simulink model "TSCLAB_Modelv_15_2020a"  (R2020a)
settings: Solver=VariableStepAuto  StartTime=0.0  StopTime=200  RelTol=1e-3
undefined symbols (not defined in the file): LF, serial
libraries: instrumentlib x3
settings Model: Creator=vasanza  LastModifiedBy=victo

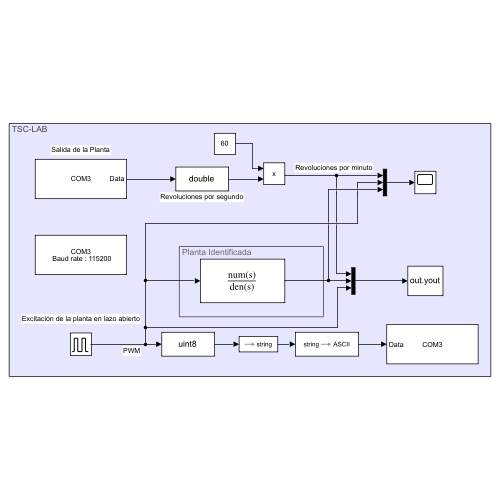
[thumbnail: Simulink's stored preview of the top-level diagram]
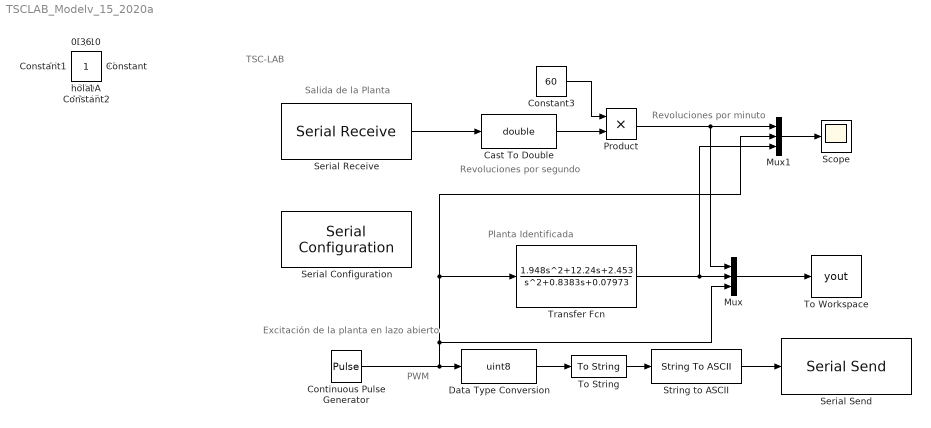
== system TSCLAB_Modelv_15_2020a ==
  note: PWM
  note: Excitación de la planta en lazo abierto
  note: Planta Identificada
  note: Revoluciones por minuto
  note: Revoluciones por segundo
  note: Salida de la Planta
  note: TSC-LAB
  Cast To Double : DataTypeConversion  OutDataTypeStr=double
  Constant3 : Constant  Value=60
  Continuous Pulse Generator : DiscretePulseGenerator  PulseType=Time based  Amplitude=255  Period=24  PulseWidth=50
  Data Type Conversion : DataTypeConversion  OutDataTypeStr=uint8
  Mux : Mux  Inputs=3
  Mux1 : Mux  Inputs=3
  Product : Product
  Scope : Scope
  Serial Configuration : instrumentlib/Serial Configuration  Priority=-200000  ObjConstructor=serial('COM3');  ComPortMenu=COM3  ComPort=COM3  BaudRate=115200  DataBits=8  Parity=none  StopBits=1  ByteOrder=LittleEndian  FlowControl=none  Timeout=10
      settings: SourceProductBaseCode=OT,IC,MT
  Serial Receive : instrumentlib/Serial Receive  ObjConstructor=serial('COM3');  ComPortMenu=COM3  ComPort=COM3  DataType=uint8  Terminator=<none>  DataSize=[1 1]  EnableBlockingMode=on  ActionDataUnavailable=Output last received value  CustomValue=0  SampleTime=0.999
      settings: SourceProductBaseCode=OT,IC,MT
  Serial Send : instrumentlib/Serial Send  ObjConstructor=serial('COM3');  ComPortMenu=COM3  ComPort=COM3  Terminator=LF ('\n')  EnableBlockingMode=on
      settings: SourceProductBaseCode=OT,IC,MT
  String to ASCII : StringToASCII
  To String : ToString
  To Workspace : ToWorkspace  VariableName=yout  SampleTime=-1
      settings: Save2DSignal=2-D array (concatenate along first dimension)
  Transfer Fcn : TransferFcn  Numerator=[1.948 12.24 2.453]  Denominator=[1 0.8383 0.07973]
  $ : Constant  IOType=siggen  Value=36
  , : Constant  IOType=siggen  Value=44
  {0,10,255,311,12345} (5 alike) : Constant  IOType=siggen
  0A : Constant  IOType=siggen  Value=10
  0D : Constant  IOType=siggen  Value=13
  13 : Constant  IOType=siggen  Value=13
  36 : Constant  IOType=siggen  Value=36
  Constant : Constant  IOType=siggen
  Constant1 : Constant  IOType=siggen
  Constant2 : Constant  IOType=siggen
  hola : Constant  IOType=siggen
  wires:
  Mux/1 -> To Workspace/1
  Transfer Fcn/1 -> Mux1/3, Mux/2
  Data Type Conversion/1 -> To String/1
  To String/1 -> String to ASCII/1
  String to ASCII/1 -> Serial Send/1
  Serial Receive/1 -> Cast To Double/1
  Mux1/1 -> Scope/1
  Continuous Pulse Generator/1 -> Data Type Conversion/1, Mux/3, Transfer Fcn/1, Mux1/2
  Cast To Double/1 -> Product/2
  Constant3/1 -> Product/1
  Product/1 -> Mux/1, Mux1/1
